simulink model "zad1"  (R2020b)
settings: Solver=FixedStepDiscrete  StartTime=0.0  StopTime=0.0  RelTol=1e-3
libraries: CPOiS_SourcesSinks x5, CPOiS_HistogramOperations x3, CPOiS_General x1
settings Model: Creator=jrybarz  LastModifiedBy=jrybarz

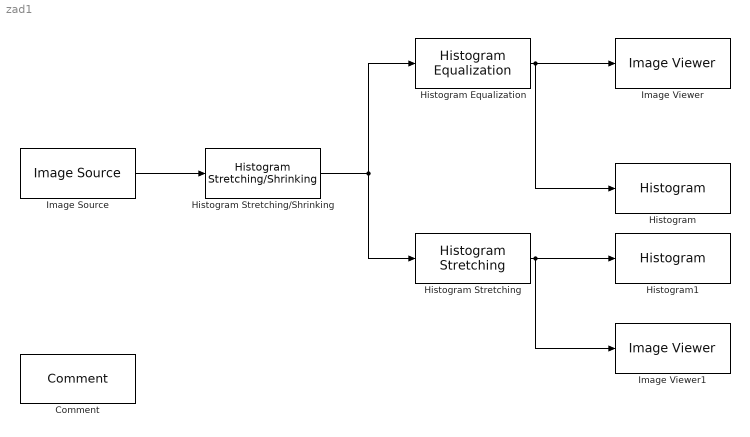
== system zad1 ==
  Comment : CPOiS_General/Comment
      settings: SourceProductName=CPOiS - Digital image and signal processing
  Histogram : CPOiS_SourcesSinks/Histogram
      settings: SourceProductName=CPOiS - Digital image and signal processing
  Histogram Stretching/Shrinking : CPOiS_HistogramOperations/Histogram Stretching//Shrinking  minimum=64  maximum=191
      settings: SourceProductName=CPOiS - Digital image and signal processing
  Histogram Equalization : CPOiS_HistogramOperations/Histogram Equalization
      settings: SourceProductName=CPOiS - Digital image and signal processing
  Histogram Stretching : CPOiS_HistogramOperations/Histogram Stretching
      settings: SourceProductName=CPOiS - Digital image and signal processing
  Histogram1 : CPOiS_SourcesSinks/Histogram
      settings: SourceProductName=CPOiS - Digital image and signal processing
  Image Source : CPOiS_SourcesSinks/Image Source  FileSelection=moon.png
      settings: SourceProductName=CPOiS - Digital image and signal processing
  Image Viewer : CPOiS_SourcesSinks/Image Viewer
      settings: SourceProductName=CPOiS - Digital image and signal processing
  Image Viewer1 : CPOiS_SourcesSinks/Image Viewer
      settings: SourceProductName=CPOiS - Digital image and signal processing
  wires:
  Histogram Stretching/Shrinking/1 -> Histogram Stretching/1, Histogram Equalization/1
  Image Source/1 -> Histogram Stretching/Shrinking/1
  Histogram Equalization/1 -> Histogram/1, Image Viewer/1
  Histogram Stretching/1 -> Image Viewer1/1, Histogram1/1
